simulink model "exp3_1"  (R2020b)
settings: Solver=VariableStepAuto  StartTime=0.0  StopTime=100  RelTol=1e-3
values from neighbouring files (symbols this model uses):
  A = [-4 1 0 0 0 0;0 -4 0 0 0 0;0 0 3 1 0 0;0 0 0 3 0 0;0 0 0 0 -1 1;0 0 0 0 0 -1]    [exp2_2.m]    (also in exp3_1.m = [-1 0 0 0;2 -3 0 0;0 0 2 0;4 -1 2 -4])
  B = [1 3;5 7;4 3;0 0;1 6;0 0]    [exp2_2.m]    (also in exp3_1.m = [0;0;1;2])
  C = [3 1 0 5 0 0;1 4 0 2 0 0]    [exp2_2.m]    (also in exp3_1.m = [3 0 1 0])
  G = [0;0;G]    [exp3_1.m]
  K1 = K1*T1    [exp3_1.m]
settings Model: Creator=86180  LastModifiedBy=CLINT
settings DataIOCC: ReturnWorkspaceOutputs=off
settings DebuggingCC: ArithmeticOperatorsInVariantConditions=warning
settings SFSimCC: SimUseLocalCustomCode=off  CustomCodeUndefinedFunction=UseInterfaceOnly
settings RTWCC: RTWUseLocalCustomCode=off
settings CodeAppCC: StateflowObjectComments=on

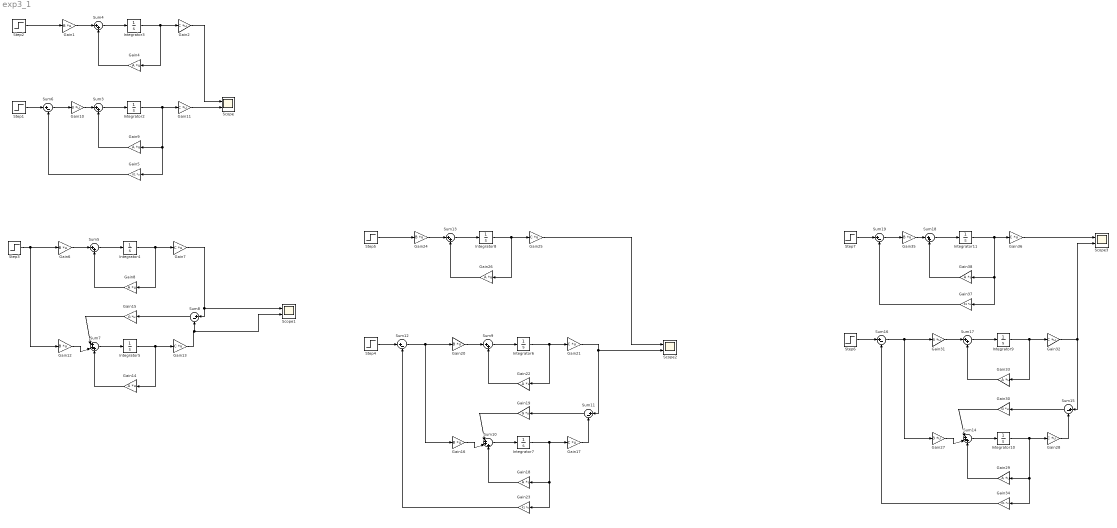
== system exp3_1 ==
  Gain{1,6,10,12,16,20,24,27,31,35} (10 alike) : Gain  Gain=B  Multiplication=Matrix(K*u)
  Gain{2,7,11,13,17,21,25,28,32,36} (10 alike) : Gain  Gain=C  Multiplication=Matrix(K*u)
  Gain{4,8..9,14,18,22,26,29,33,38} (10 alike) : Gain  Gain=A  Multiplication=Matrix(K*u)
  Gain15 : Gain  Gain=G  Multiplication=Matrix(K*u)
  Gain19 : Gain  Gain=G  Multiplication=Matrix(K*u)
  Gain{5,23,34,37} (4 alike) : Gain  Gain=K1  Multiplication=Matrix(K*u)
  Gain30 : Gain  Gain=G  Multiplication=Matrix(K*u)
  Integrator10 : Integrator  InitialCondition=[0;0;2;1]
  Integrator{2..4,6,8..9,11} (7 alike) : Integrator
  Integrator5 : Integrator  InitialCondition=[0;0;2;1]
  Integrator7 : Integrator  InitialCondition=[0;0;2;1]
  Scope{,1..3} (4 alike) : Scope  NumInputPorts=2
  Step{1..7} (7 alike) : Step  SampleTime=0
  Sum10 : Sum  Inputs=|+++
  Sum{6,8,11..12,15..16,19} (7 alike) : Sum  Inputs=|+-
  Sum{3..5,9,13,17..18} (7 alike) : Sum  Inputs=|++
  Sum14 : Sum  Inputs=|+++
  Sum7 : Sum  Inputs=|+++
  wires:
  Gain10/1 -> Sum3/1
  Sum3/1 -> Integrator2/1
  Gain11/1 -> Scope/2
  Integrator2/1 -> Gain11/1, Gain9/1, Gain5/1
  Gain9/1 -> Sum3/2
  Gain4/1 -> Sum4/2
  Integrator3/1 -> Gain4/1, Gain2/1
  Step2/1 -> Gain1/1
  Sum4/1 -> Integrator3/1
  Gain1/1 -> Sum4/1
  Gain2/1 -> Scope/1
  Step1/1 -> Sum6/1
  Sum6/1 -> Gain10/1
  Gain5/1 -> Sum6/2
  Gain6/1 -> Sum5/1
  Gain8/1 -> Sum5/2
  Sum5/1 -> Integrator4/1
  Integrator4/1 -> Gain8/1, Gain7/1
  Sum7/1 -> Integrator5/1
  Gain14/1 -> Sum7/3
  Integrator5/1 -> Gain14/1, Gain13/1
  Gain12/1 -> Sum7/2
  Step3/1 -> Gain12/1, Gain6/1
  Gain13/1 -> Scope1/2, Sum8/2
  Gain7/1 -> Scope1/1, Sum8/1
  Sum8/1 -> Gain15/1
  Gain15/1 -> Sum7/1
  Gain19/1 -> Sum10/1
  Gain22/1 -> Sum9/2
  Sum9/1 -> Integrator6/1
  Integrator6/1 -> Gain22/1, Gain21/1
  Gain20/1 -> Sum9/1
  Gain21/1 -> Scope2/2, Sum11/1
  Sum10/1 -> Integrator7/1
  Gain18/1 -> Sum10/3
  Gain16/1 -> Sum10/2
  Gain17/1 -> Sum11/2
  Sum11/1 -> Gain19/1
  Integrator7/1 -> Gain23/1, Gain18/1, Gain17/1
  Step4/1 -> Sum12/1
  Sum12/1 -> Gain16/1, Gain20/1
  Gain23/1 -> Sum12/2
  Gain24/1 -> Sum13/1
  Step5/1 -> Gain24/1
  Gain26/1 -> Sum13/2
  Sum13/1 -> Integrator8/1
  Integrator8/1 -> Gain26/1, Gain25/1
  Gain25/1 -> Scope2/1
  Gain28/1 -> Sum15/2
  Integrator10/1 -> Gain34/1, Gain29/1, Gain28/1
  Sum15/1 -> Gain30/1
  Sum14/1 -> Integrator10/1
  Gain29/1 -> Sum14/3
  Step6/1 -> Sum16/1
  Gain32/1 -> Sum15/1, Scope3/2
  Gain27/1 -> Sum14/2
  Gain31/1 -> Sum17/1
  Integrator9/1 -> Gain33/1, Gain32/1
  Gain33/1 -> Sum17/2
  Gain30/1 -> Sum14/1
  Gain34/1 -> Sum16/2
  Sum17/1 -> Integrator9/1
  Sum16/1 -> Gain27/1, Gain31/1
  Gain36/1 -> Scope3/1
  Sum19/1 -> Gain35/1
  Gain37/1 -> Sum19/2
  Gain35/1 -> Sum18/1
  Gain38/1 -> Sum18/2
  Integrator11/1 -> Gain36/1, Gain38/1, Gain37/1
  Step7/1 -> Sum19/1
  Sum18/1 -> Integrator11/1
